simulink model "nir_d2"  (R2022a)
settings: Solver=ode15s  StartTime=0.0  StopTime=30  RelTol=1e-3
undefined symbols (not defined in the file): alpha, beta, c, dY_init, flux_init, g, Gamma, gamma_lam1, gamma_lam2, gamma_nu, gamma_Y, k, k1, k2, m, nu1, nu2, R, R_a, Y_init
settings Model: Creator=Ochir  LastModifiedBy=Ochir

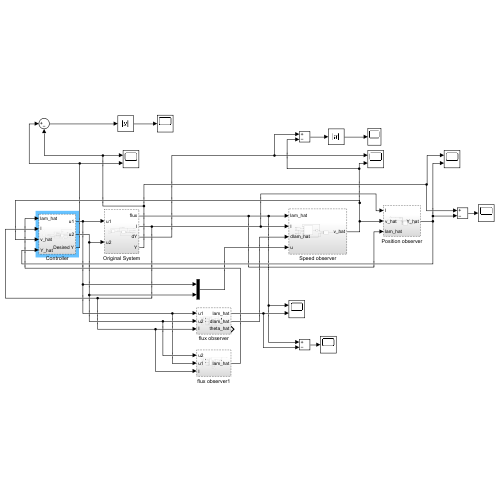
[thumbnail: Simulink's stored preview of the top-level diagram]
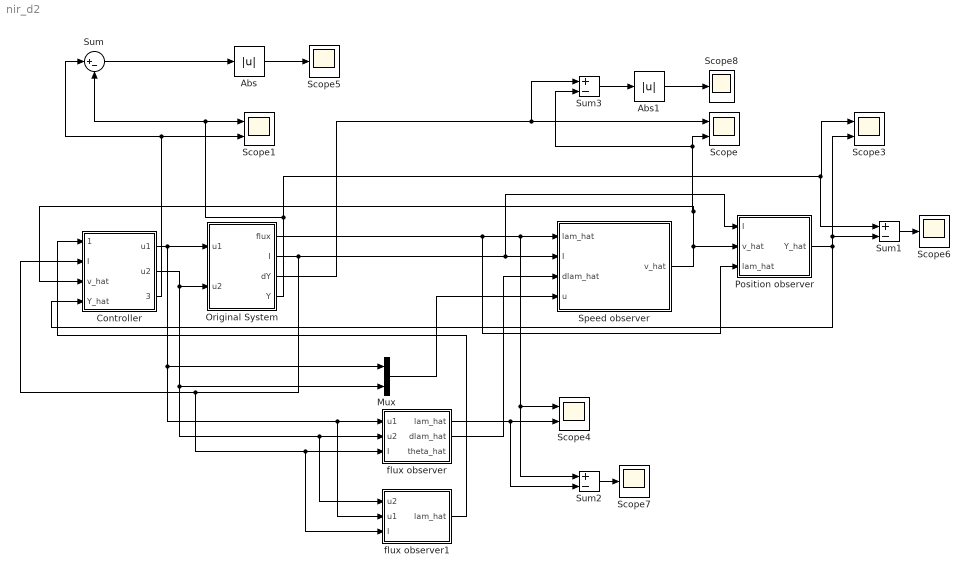
== system nir_d2 ==
  Abs : Abs  SaturateOnIntegerOverflow=off
  Abs1 : Abs  SaturateOnIntegerOverflow=off
  Controller : Subsystem  Priority=4
      settings: MinAlgLoopOccurrences=on
  Mux : Mux  Inputs=2
  Original System : Subsystem
      settings: MinAlgLoopOccurrences=on
  Position observer : Subsystem
      settings: MinAlgLoopOccurrences=on
  Scope{,1,3..4} (4 alike) : Scope  NumInputPorts=2
  Scope{5..8} (4 alike) : Scope
  Speed observer : Subsystem
      settings: MinAlgLoopOccurrences=on
  Sum : Sum  Inputs=|+-
  Sum1 : Sum  Inputs=+-
  Sum2 : Sum  Inputs=+-
  Sum3 : Sum  Inputs=+-
  flux observer : Subsystem
      settings: MinAlgLoopOccurrences=on
  flux observer1 : Subsystem
      settings: MinAlgLoopOccurrences=on
  wires:
  Controller/2(u2) -> flux observer1/1(u2), flux observer/2(u2), Mux/2, Original System/2(u2)
  Sum3/1 -> Abs1/1
  Sum2/1 -> Scope7/1
  Speed observer/1(v_hat) -> Controller/3(v_hat), Sum3/2, Scope/2, Position observer/2(v_hat)
  flux observer/2(dlam_hat) -> Speed observer/3(dlam_hat)
  flux observer/1(lam_hat) -> Sum2/2, Scope4/2
  Position observer/1(Y_hat) -> Controller/4(Y_hat), Sum1/2, Scope3/2
  Original System/2(I) -> Position observer/1(I), Speed observer/2(I), flux observer1/3(I), flux observer/3(I), Controller/2(I)
  flux observer1/1(lam_hat) -> Controller/1(lam_hat)
  Controller/1(u1) -> flux observer1/2(u1), flux observer/1(u1), Mux/1, Original System/1(u1)
  Abs/1 -> Scope5/1
  Original System/4(Y) -> Scope1/1, Sum/2, Sum1/1, Scope3/1
  Original System/1(flux) -> Position observer/3(lam_hat), Sum2/1, Scope4/1, Speed observer/1(lam_hat)
  Sum1/1 -> Scope6/1
  Controller/3(Desired Y) -> Scope1/2, Sum/1
  Sum/1 -> Abs/1
  Mux/1 -> Speed observer/4(u)
  Original System/3(dY) -> Sum3/1, Scope/1
  Abs1/1 -> Scope8/1

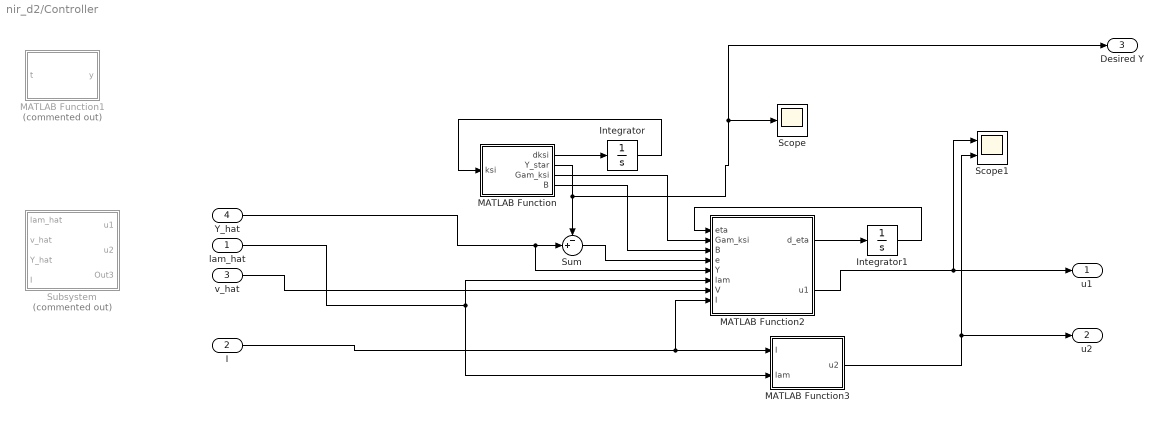
== system nir_d2/Controller ==
  lam_hat : Inport
  I : Inport  Port=2
  v_hat : Inport  Port=3
  Y_hat : Inport  Port=4
  Integrator : Integrator  InitialCondition=[0.01; -0.01]
  Integrator1 : Integrator  InitialCondition=[0.01; -0.01]
  MATLAB Function : MATLAB Function  TreatAsAtomicUnit=on
  MATLAB Function1 : MATLAB Function  Commented=on  TreatAsAtomicUnit=on
  MATLAB Function2 : MATLAB Function  TreatAsAtomicUnit=on
  MATLAB Function3 : MATLAB Function  TreatAsAtomicUnit=on
  Scope : Scope
  Scope1 : Scope  NumInputPorts=2
  Subsystem : Subsystem  Commented=on
  Sum : Sum  Inputs=-+|
  u1 : Outport
  u2 : Outport  Port=2
  Desired Y : Outport  Port=3
  wires:
  Integrator1/1 -> MATLAB Function2/1(eta)
  lam_hat/1 -> MATLAB Function3/2(lam), MATLAB Function2/6(lam)
  MATLAB Function2/1(d_eta) -> Integrator1/1
  Sum/1 -> MATLAB Function2/4(e)
  Y_hat/1 -> MATLAB Function2/5(Y), Sum/2
  Integrator/1 -> MATLAB Function/1(ksi)
  MATLAB Function/3(Gam_ksi) -> MATLAB Function2/2(Gam_ksi)
  MATLAB Function/1(dksi) -> Integrator/1
  MATLAB Function/2(Y_star) -> Sum/1, Desired Y/1, Scope/1
  MATLAB Function3/1(u2) -> u2/1, Scope1/2
  MATLAB Function2/2(u1) -> u1/1, Scope1/1
  MATLAB Function/4(B) -> MATLAB Function2/3(B)
  v_hat/1 -> MATLAB Function2/7(V)
  I/1 -> MATLAB Function2/8(I), MATLAB Function3/1(I)

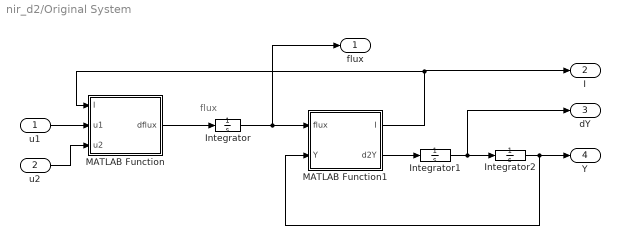
== system nir_d2/Original System ==
  note: flux
  u1 : Inport
  u2 : Inport  Port=2
  Integrator : Integrator  InitialCondition=flux_init  UpperSaturationLimit=1e12  LowerSaturationLimit=-1e12
  Integrator1 : Integrator  InitialCondition=dY_init  UpperSaturationLimit=1e12  LowerSaturationLimit=-1e12
  Integrator2 : Integrator  InitialCondition=Y_init  UpperSaturationLimit=1e12  LowerSaturationLimit=-1e12
  MATLAB Function : MATLAB Function  Priority=0
  MATLAB Function1 : MATLAB Function  Priority=0
  flux : Outport
  I : Outport  Port=2
  dY : Outport  Port=3
  Y : Outport  Port=4
  wires:
  Integrator/1 -> flux/1, MATLAB Function1/1(flux)
  u1/1 -> MATLAB Function/2(u1)
  u2/1 -> MATLAB Function/3(u2)
  MATLAB Function/1(dflux) -> Integrator/1
  MATLAB Function1/2(d2Y) -> Integrator1/1
  Integrator1/1 -> dY/1, Integrator2/1
  Integrator2/1 -> Y/1, MATLAB Function1/2(Y)
  MATLAB Function1/1(I) -> I/1, MATLAB Function/1(I)

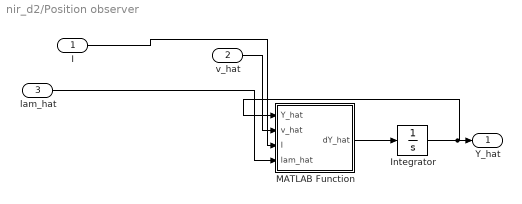
== system nir_d2/Position observer ==
  I : Inport
  v_hat : Inport  Port=2
  lam_hat : Inport  Port=3
  Integrator : Integrator  UpperSaturationLimit=1e12  LowerSaturationLimit=-1e12
  MATLAB Function : MATLAB Function
  Y_hat : Outport
  wires:
  Integrator/1 -> MATLAB Function/1(Y_hat), Y_hat/1
  lam_hat/1 -> MATLAB Function/4(lam_hat)
  I/1 -> MATLAB Function/3(I)
  v_hat/1 -> MATLAB Function/2(v_hat)
  MATLAB Function/1(dY_hat) -> Integrator/1

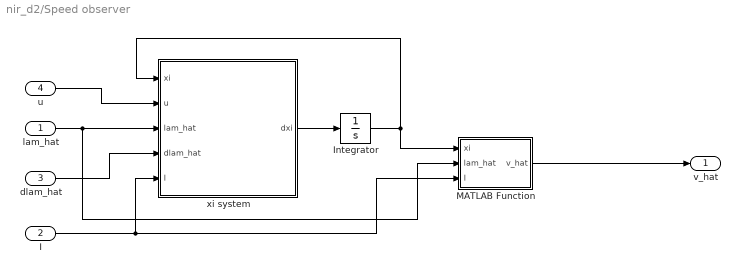
== system nir_d2/Speed observer ==
  lam_hat : Inport
  I : Inport  Port=2
  dlam_hat : Inport  Port=3
  u : Inport  Port=4
  Integrator : Integrator  UpperSaturationLimit=1e12  LowerSaturationLimit=-1e12
  MATLAB Function : MATLAB Function
  xi system : MATLAB Function
  v_hat : Outport
  wires:
  dlam_hat/1 -> xi system/4(dlam_hat)
  I/1 -> xi system/5(I), MATLAB Function/3(I)
  Integrator/1 -> xi system/1(xi), MATLAB Function/1(xi)
  xi system/1(dxi) -> Integrator/1
  MATLAB Function/1(v_hat) -> v_hat/1
  u/1 -> xi system/2(u)
  lam_hat/1 -> MATLAB Function/2(lam_hat), xi system/3(lam_hat)

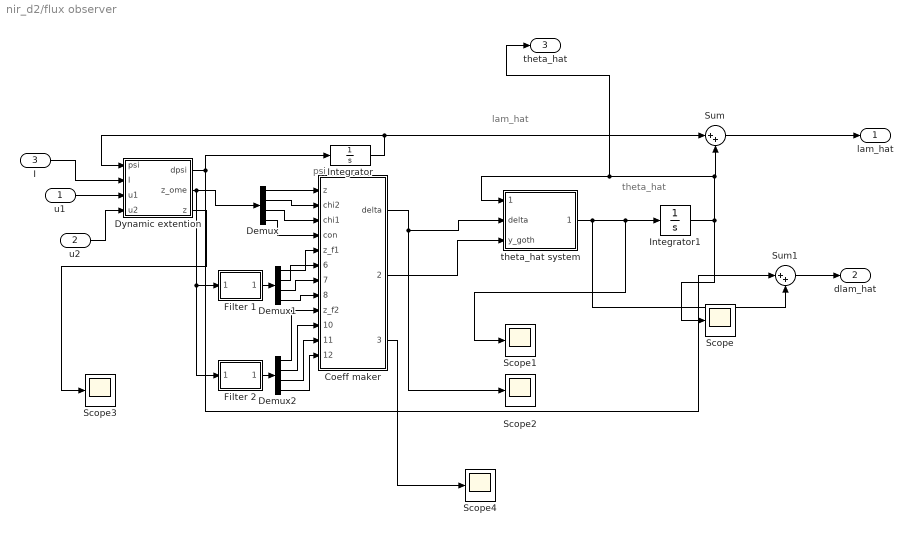
== system nir_d2/flux observer ==
  note: lam_hat
  note: theta_hat
  note: psi
  u1 : Inport
  u2 : Inport  Port=2
  I : Inport  Port=3
  Coeff maker : MATLAB Function  Priority=4
  Demux : Demux
  Demux1 : Demux
  Demux2 : Demux
  Dynamic extention : MATLAB Function  Priority=0
  Filter 1 : Subsystem  Priority=0
  Filter 2 : Subsystem  Priority=1
  Integrator : Integrator  InitialCondition=[0;0]  UpperSaturationLimit=1e12  LowerSaturationLimit=-1e12
  Integrator1 : Integrator  InitialCondition=[0;0]  UpperSaturationLimit=1e12  LowerSaturationLimit=-1e12
  Scope{,1..4} (5 alike) : Scope
  Sum : Sum  Priority=8  Inputs=|++
  Sum1 : Sum  Priority=7  Inputs=|++
  theta_hat system : MATLAB Function  Priority=5
  lam_hat : Outport
  dlam_hat : Outport  Port=2
  theta_hat : Outport  Port=3
  wires:
  u2/1 -> Dynamic extention/4(u2)
  Integrator/1 -> Dynamic extention/1(psi), Sum/1
  u1/1 -> Dynamic extention/3(u1)
  Sum/1 -> lam_hat/1
  Sum1/1 -> dlam_hat/1
  Dynamic extention/1(dpsi) -> Sum1/1, Integrator/1
  Dynamic extention/2(z_ome) -> Demux/1, Filter 2/1(z_ome), Filter 1/1(z_ome)
  I/1 -> Dynamic extention/2(I)
  theta_hat system/1(dtheta_hat) -> Sum1/2, Scope1/1, Integrator1/1
  Coeff maker/2(y_goth) -> theta_hat system/3(y_goth)
  Coeff maker/1(delta) -> Scope2/1, theta_hat system/2(delta)
  Integrator1/1 -> Scope/1, theta_hat system/1(theta_hat), theta_hat/1, Sum/2
  Demux/1 -> Coeff maker/1(z)
  Demux/2 -> Coeff maker/2(chi2)
  Demux/3 -> Coeff maker/3(chi1)
  Demux/4 -> Coeff maker/4(con)
  Filter 1/1(Output) -> Demux1/1
  Demux1/1 -> Coeff maker/5(z_f1)
  Demux1/2 -> Coeff maker/6(chi2_f1)
  Demux1/3 -> Coeff maker/7(chi1_f1)
  Demux1/4 -> Coeff maker/8(con_f1)
  Filter 2/1(Output) -> Demux2/1
  Demux2/1 -> Coeff maker/9(z_f2)
  Demux2/2 -> Coeff maker/10(chi2_f2)
  Demux2/3 -> Coeff maker/11(chi1_f2)
  Demux2/4 -> Coeff maker/12(con_f2)
  Dynamic extention/3(z) -> Scope3/1
  Coeff maker/3(rang_Omega) -> Scope4/1

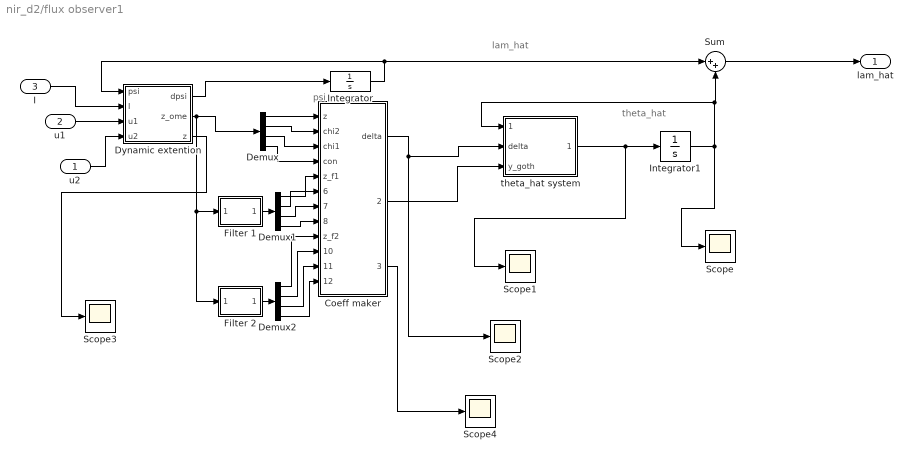
== system nir_d2/flux observer1 ==
  note: lam_hat
  note: theta_hat
  note: psi
  u2 : Inport
  u1 : Inport  Port=2
  I : Inport  Port=3
  Coeff maker : MATLAB Function  Priority=4
  Demux : Demux
  Demux1 : Demux
  Demux2 : Demux
  Dynamic extention : MATLAB Function  Priority=0
  Filter 1 : Subsystem  Priority=0
  Filter 2 : Subsystem  Priority=1
  Integrator : Integrator  InitialCondition=[0;0]  UpperSaturationLimit=1e12  LowerSaturationLimit=-1e12
  Integrator1 : Integrator  InitialCondition=[0;0]  UpperSaturationLimit=1e12  LowerSaturationLimit=-1e12
  Scope{,1..4} (5 alike) : Scope
  Sum : Sum  Priority=8  Inputs=|++
  theta_hat system : MATLAB Function  Priority=5
  lam_hat : Outport
  wires:
  u2/1 -> Dynamic extention/4(u2)
  Integrator/1 -> Dynamic extention/1(psi), Sum/1
  u1/1 -> Dynamic extention/3(u1)
  Sum/1 -> lam_hat/1
  Dynamic extention/1(dpsi) -> Integrator/1
  Dynamic extention/2(z_ome) -> Demux/1, Filter 2/1(z_ome), Filter 1/1(z_ome)
  I/1 -> Dynamic extention/2(I)
  theta_hat system/1(dtheta_hat) -> Scope1/1, Integrator1/1
  Coeff maker/2(y_goth) -> theta_hat system/3(y_goth)
  Coeff maker/1(delta) -> Scope2/1, theta_hat system/2(delta)
  Integrator1/1 -> Scope/1, theta_hat system/1(theta_hat), Sum/2
  Demux/1 -> Coeff maker/1(z)
  Demux/2 -> Coeff maker/2(chi2)
  Demux/3 -> Coeff maker/3(chi1)
  Demux/4 -> Coeff maker/4(con)
  Filter 1/1(Output) -> Demux1/1
  Demux1/1 -> Coeff maker/5(z_f1)
  Demux1/2 -> Coeff maker/6(chi2_f1)
  Demux1/3 -> Coeff maker/7(chi1_f1)
  Demux1/4 -> Coeff maker/8(con_f1)
  Filter 2/1(Output) -> Demux2/1
  Demux2/1 -> Coeff maker/9(z_f2)
  Demux2/2 -> Coeff maker/10(chi2_f2)
  Demux2/3 -> Coeff maker/11(chi1_f2)
  Demux2/4 -> Coeff maker/12(con_f2)
  Dynamic extention/3(z) -> Scope3/1
  Coeff maker/3(rang_Omega) -> Scope4/1

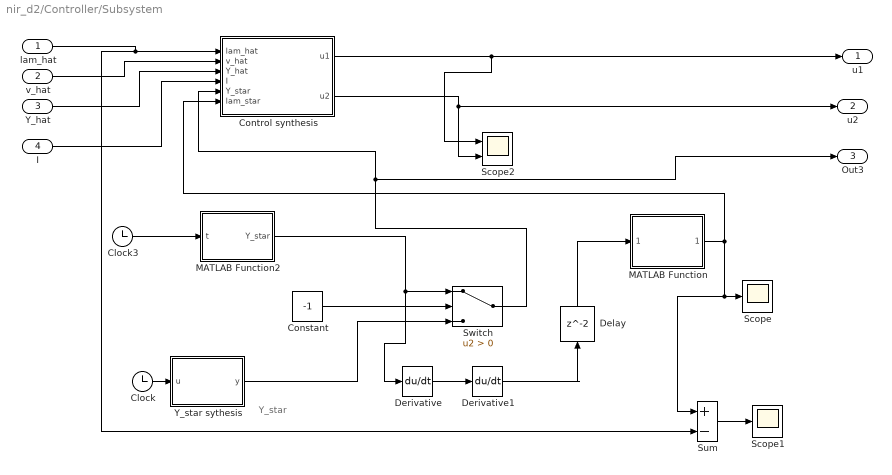
== system nir_d2/Controller/Subsystem ==
  note: Y_star
  lam_hat : Inport
  v_hat : Inport  Port=2
  Y_hat : Inport  Port=3
  I : Inport  Port=4
  Clock : Clock
  Clock3 : Clock
  Constant : Constant  Value=-1
  Control synthesis : MATLAB Function  Priority=1
  Delay : Delay
  Derivative : Derivative
  Derivative1 : Derivative
  MATLAB Function : MATLAB Function  TreatAsAtomicUnit=on
  MATLAB Function2 : MATLAB Function  TreatAsAtomicUnit=on
  Scope : Scope
  Scope1 : Scope
  Scope2 : Scope  NumInputPorts=2
  Sum : Sum  Inputs=+-
  Switch : Switch  Criteria=u2 > Threshold  SaturateOnIntegerOverflow=off  InputSameDT=off
  Y_star sythesis : MATLAB Function  Priority=0
  u1 : Outport
  u2 : Outport  Port=2
  Out3 : Outport  Port=3
  wires:
  MATLAB Function2/1(Y_star) -> Derivative/1, Switch/1
  MATLAB Function/1(lambda_star) -> Scope/1, Sum/1, Control synthesis/6(lam_star)
  lam_hat/1 -> Control synthesis/1(lam_hat), Sum/2
  Clock/1 -> Y_star sythesis/1(u)
  Y_star sythesis/1(y) -> Switch/3
  Switch/1 -> Out3/1, Control synthesis/5(Y_star)
  Constant/1 -> Switch/2
  Derivative/1 -> Derivative1/1
  Clock3/1 -> MATLAB Function2/1(t)
  Control synthesis/2(u2) -> u2/1, Scope2/2
  Control synthesis/1(u1) -> u1/1, Scope2/1
  Derivative1/1 -> Delay/1
  Sum/1 -> Scope1/1
  Delay/1 -> MATLAB Function/1(d2Y_star)
  v_hat/1 -> Control synthesis/2(v_hat)
  Y_hat/1 -> Control synthesis/3(Y_hat)
  I/1 -> Control synthesis/4(I)

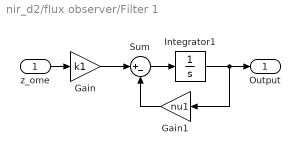
== system nir_d2/flux observer/Filter 1 ==
  z_ome : Inport
  Gain : Gain  Gain=k1
  Gain1 : Gain  Gain=nu1
  Integrator1 : Integrator  InitialCondition=[0; 0; 0; 0]  UpperSaturationLimit=1e12  LowerSaturationLimit=-1e12
  Sum : Sum  Inputs=|+-
  Output : Outport
  wires:
  Sum/1 -> Integrator1/1
  Gain/1 -> Sum/1
  Integrator1/1 -> Output/1, Gain1/1
  Gain1/1 -> Sum/2
  z_ome/1 -> Gain/1

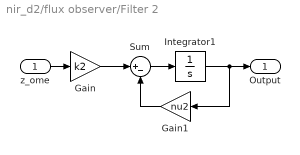
== system nir_d2/flux observer/Filter 2 ==
  z_ome : Inport
  Gain : Gain  Gain=k2
  Gain1 : Gain  Gain=nu2
  Integrator1 : Integrator  InitialCondition=[0; 0; 0; 0]  UpperSaturationLimit=1e12  LowerSaturationLimit=-1e12
  Sum : Sum  Inputs=|+-
  Output : Outport
  wires:
  Sum/1 -> Integrator1/1
  Gain/1 -> Sum/1
  Integrator1/1 -> Output/1, Gain1/1
  Gain1/1 -> Sum/2
  z_ome/1 -> Gain/1

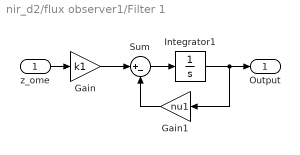
== system nir_d2/flux observer1/Filter 1 ==
  z_ome : Inport
  Gain : Gain  Gain=k1
  Gain1 : Gain  Gain=nu1
  Integrator1 : Integrator  InitialCondition=[0; 0; 0; 0]  UpperSaturationLimit=1e12  LowerSaturationLimit=-1e12
  Sum : Sum  Inputs=|+-
  Output : Outport
  wires:
  Sum/1 -> Integrator1/1
  Gain/1 -> Sum/1
  Integrator1/1 -> Output/1, Gain1/1
  Gain1/1 -> Sum/2
  z_ome/1 -> Gain/1

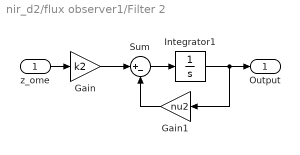
== system nir_d2/flux observer1/Filter 2 ==
  z_ome : Inport
  Gain : Gain  Gain=k2
  Gain1 : Gain  Gain=nu2
  Integrator1 : Integrator  InitialCondition=[0; 0; 0; 0]  UpperSaturationLimit=1e12  LowerSaturationLimit=-1e12
  Sum : Sum  Inputs=|+-
  Output : Outport
  wires:
  Sum/1 -> Integrator1/1
  Gain/1 -> Sum/1
  Integrator1/1 -> Output/1, Gain1/1
  Gain1/1 -> Sum/2
  z_ome/1 -> Gain/1

== matlab function nir_d2/Controller/Subsystem/Control synthesis ==
  data: lam_hat input size=[2,1]; u1 output size=1; v_hat input size=1; Y_hat input size=1; I input size=[2,1]; Y_star input size=1; u2 output size=1; R parameter; k parameter; alpha parameter; beta parameter; Gamma parameter; m parameter; R_a parameter; lam_star input
function [u1, u2] = fcn(lam_hat, v_hat, Y_hat, I, Y_star, R, k, alpha, beta, Gamma, m, R_a, lam_star)
    lam_wave = [0;0];
    lam_wave(1) = (lam_hat(1) - lam_star(1));
    lam_wave(2) = lam_hat(2) - lam_star(2);
    Y_wave = (Y_hat - Y_star);
    u1 = R*I(1) - R/2/k/alpha*(lam_hat(1)^2 - lam_star(1)^2) - (R/alpha+alpha*R_a)*...
          Gamma*(1/alpha*lam_wave(1) + Y_wave + R_a*m*v_hat) - alpha*v_hat;
    
    u2 = R*I(2) - R/2/k/beta*(lam_hat(2)^2 - lam_star(2)^2) + beta*R_a*...
          Gamma*(1/alpha*lam_wave(1) + Y_wave + R_a*m*v_hat) + beta*v_hat;

== matlab function nir_d2/flux observer1/Dynamic extention ==
  data: psi input size=[2,1]; I input size=[2,1]; dpsi output size=[2, 1]; u1 input; u2 input; g parameter; c parameter; m parameter; k parameter; R parameter; z_ome output; z output size=1
function [dpsi, z_ome, z]  = fcn(psi, I, u1, u2, g, c, m, k, R)
    u = [u1; u2];
    dpsi = -R*I + u;
    z = -I(1)*psi(2)-I(2)*psi(1) + 2*c/k*psi(1)*psi(2);
    chi = I - 2*c/k*psi;
    
    z_ome = [z; chi(2); chi(1); -(2*c/k)];

== matlab function nir_d2/flux observer1/theta_hat system ==
  data: theta_hat input; delta input; y_goth input; dtheta_hat output size=[2, 1]; gamma_lam1 parameter; gamma_lam2 parameter
function dtheta_hat = fcn(theta_hat, delta, y_goth, gamma_lam1, gamma_lam2)
 
    dtheta_hat = [gamma_lam1*delta*(y_goth(1) - delta*theta_hat(1)); ...
                gamma_lam2*delta*(y_goth(2) - delta*theta_hat(2))];

== matlab function nir_d2/Controller/Subsystem/MATLAB Function ==
  data: d2Y_star input; lambda_star output; k parameter; m parameter; g parameter
function lambda_star = fcn(d2Y_star, k, m, g)

    lambda_star = [0; 0];
    lambda_star(2) = 1;
    lambda_star(1) = sqrt(2*k*m*(g+0) + 1^2);
    %lambda_star(1) = sqrt(2*k*m*g + 1);

== matlab function nir_d2/Original System/MATLAB Function ==
  data: I input; dflux output size=[2 1]; u1 input; u2 input; R parameter
function dflux  = fcn(I, u1, u2, R)
    dflux = [-R*I(1) + u1; -R*I(2) + u2];

== matlab function nir_d2/Speed observer/xi system ==
  data: xi input; dxi output size=1; u input; lam_hat input; dlam_hat input; I input; g parameter; k parameter; m parameter; gamma_nu parameter; R parameter
function dxi = fcn(xi, u, lam_hat, dlam_hat, I, g, k, m, gamma_nu, R)
    dlam = -R*I + u;
    dxi = -gamma_nu*(norm(lam_hat)^2)*(xi - gamma_nu*k*( I(1)*lam_hat(1) -I(2)*lam_hat(2)))...
         + gamma_nu*k*I(1)*(dlam(1) + dlam_hat(1)) - gamma_nu*k*I(2)*(dlam(2) + dlam_hat(2))...
          + 1/2/k/m*((lam_hat(1))^2 - (lam_hat(2))^2) - g;

    

    %dxi = -gamma_nu*(norm(lam)^2*v_hat - 2*k*(I(1)*dlam(1) - I(2)*dlam(2))) + 1/2/k/m*(lam(1)^2-lam(2)^2-2*k*m*g);

== matlab function nir_d2/Position observer/MATLAB Function ==
  data: Y_hat input; dY_hat output size=1; v_hat input; I input; lam_hat input; gamma_Y parameter; k parameter; c parameter
function dY_hat = fcn(Y_hat, v_hat, I, lam_hat, gamma_Y, k, c)

    dY_hat = v_hat - gamma_Y*(norm(lam_hat)^2*Y_hat + (k*I(1) - c*lam_hat(1))*lam_hat(1) ...
              - (k*I(2) - c*lam_hat(2))*lam_hat(2));

== matlab function nir_d2/Controller/Subsystem/Y_star sythesis ==
  data: u input; y output
function y = fcn(u)
    f = 0;
    if (u>=0) && (u<1)
        f = 0.001;
    end
    if (u>=1) && (u<2)
        f = 0.002;
    end
    if (u>=2) && (u<3)
        f = -0.001;
    end
    if (u>=3) && (u<4)
        f = 0.001;
    end
    if (u>=4) && (u<5)
        f = 0.003;
    end
    if (u>=5)
        f = 0.001;
    end
    y = f;

== matlab function nir_d2/Speed observer/MATLAB Function ==
  data: xi input; v_hat output; lam_hat input; I input; gamma_nu parameter; k parameter
function v_hat = fcn(xi, lam_hat, I, gamma_nu, k)

    v_hat = xi - gamma_nu*k*(I(1)*lam_hat(1) - I(2)*lam_hat(2));

== matlab function nir_d2/Controller/MATLAB Function1 ==
  data: t input; y output
function y = fcn(t)

y = -0.005*sin(0.5*t) - 0.05*sin(t) + 0.1575*sin(1.5*t);

== matlab function nir_d2/Original System/MATLAB Function1 ==
  data: I output; flux input; g parameter; m parameter; k parameter; d2Y output; Y input; c parameter
function [I, d2Y]  = fcn(flux, g, m, k, Y, c)
    lam1 = flux(1);
    lam2 = flux(2);
    d2Y = 1/2/k/m*(lam1.^2-lam2.^2) - g;
    I = [1/k*(c - Y)*lam1; 1/k*(c + Y)*lam2];

== matlab function nir_d2/Controller/Subsystem/MATLAB Function2 ==
  data: t input; Y_star output
function Y_star = fcn(t)

Y_star = 0.02*sin(0.5*t) + 0.05*sin(t) - 0.07*sin(1.5*t);

== matlab function nir_d2/Controller/MATLAB Function ==
  data: ksi input; dksi output; Y_star output; Gam_ksi output; B output
function [dksi, Y_star, Gam_ksi, B] = fcn(ksi)

Gam_ksi = [0 2; -2 0];
%Gam_ksi = -eye(2);
B = [1; 1];
H_ksi = [1 1];
dksi = Gam_ksi*ksi;
Y_star = H_ksi*ksi;

== matlab function nir_d2/Controller/MATLAB Function2 ==
  data: eta input; Gam_ksi input; B input; e input; d_eta output; Y input; lam input size=[2, 1]; V input; R parameter; I input; u1 output; k parameter; c parameter
function [d_eta, u1] = fcn(eta, Gam_ksi, B, e, Y, lam, V, R, I, k, c)
%B = [1; 1];
d_eta = Gam_ksi*eta + B*e;

k1 = 500; % 3000 %
k_eta = 300*[1 1]; % 0.01*[1 -1]
k2 = -300; % -10 or -20
k3 = R/k*(c-Y);
u1 = k1*e + k_eta*eta - k2*V - k3*lam(2);
%k1_2 = 10;
%k_eta_2 = 0.001*[1 -1];
%k2_2 = 100;
%k3_2 = R/k*(c+Y);
%u2 = k1_2*e + k_eta_2*eta - k2_2*V - k3_2*lam(1);

== matlab function nir_d2/Controller/MATLAB Function3 ==
  data: I input size=[2, 1]; u2 output; R parameter; lam input
function u2 = fcn(I, R, lam)

u2 = I(2)*R + (2 - lam(2));

== matlab function nir_d2/flux observer1/Coeff maker ==
  data: z input; chi2 input; chi1 input; con input; delta output size=1; z_f1 input; chi2_f1 input; chi1_f1 input; con_f1 input; z_f2 input; chi2_f2 input; y_goth output size=[3, 1]; chi1_f2 input; con_f2 input; rang_Omega output
function [delta, y_goth, rang_Omega] = fcn(z, chi2, chi1, con, z_f1, chi2_f1, chi1_f1, con_f1, z_f2, chi2_f2, chi1_f2, con_f2)
    
    Z = [z; z_f1; z_f2];
    Omega = [chi2, chi1, con; chi2_f1, chi1_f1, con_f1; chi2_f2, chi1_f2, con_f2];
    delta = det(Omega);
    adj = eye(3, 3);

    adj(1, 1) = det([Omega(2, 2) Omega(2, 3); Omega(3, 2) Omega(3, 3)]);
    adj(1, 2) = -det([Omega(2, 1) Omega(2, 3); Omega(3, 1) Omega(3, 3)]);
    adj(1, 3) = det([Omega(2, 1) Omega(2, 2); Omega(3, 1) Omega(3, 2)]);

    adj(2, 1) = -det([Omega(1, 2) Omega(1, 3); Omega(3, 2) Omega(3, 3)]);
    adj(2, 2) = det([Omega(1, 1) Omega(1, 3); Omega(3, 1) Omega(3, 3)]);
    adj(2, 3) = -det([Omega(1, 1) Omega(1, 2); Omega(3, 1) Omega(3, 2)]);

    adj(3, 1) = det([Omega(1, 2) Omega(1, 3); Omega(2, 2) Omega(2, 3)]);
    adj(3, 2) = -det([Omega(1, 1) Omega(1, 3); Omega(2, 1) Omega(2, 3)]);
    adj(3, 3) = det([Omega(1, 1) Omega(1, 2); Omega(2, 1) Omega(2, 2)]);

    adj = adj';

    y_goth = adj*Z;

    %if norm(delta) < 1e-12
    %    delta = 0;
    %end
    rang_Omega = rank(Omega); 
    %should_be_diag = Omega*adj
    %delta

== matlab function nir_d2/flux observer/Coeff maker ==
  data: z input; chi2 input; chi1 input; con input; delta output size=1; z_f1 input; chi2_f1 input; chi1_f1 input; con_f1 input; z_f2 input; chi2_f2 input; y_goth output size=[3, 1]; chi1_f2 input; con_f2 input; rang_Omega output
function [delta, y_goth, rang_Omega] = fcn(z, chi2, chi1, con, z_f1, chi2_f1, chi1_f1, con_f1, z_f2, chi2_f2, chi1_f2, con_f2)
    
    Z = [z; z_f1; z_f2];
    Omega = [chi2, chi1, con; chi2_f1, chi1_f1, con_f1; chi2_f2, chi1_f2, con_f2];
    delta = det(Omega);
    adj = eye(3, 3);

    adj(1, 1) = det([Omega(2, 2) Omega(2, 3); Omega(3, 2) Omega(3, 3)]);
    adj(1, 2) = -det([Omega(2, 1) Omega(2, 3); Omega(3, 1) Omega(3, 3)]);
    adj(1, 3) = det([Omega(2, 1) Omega(2, 2); Omega(3, 1) Omega(3, 2)]);

    adj(2, 1) = -det([Omega(1, 2) Omega(1, 3); Omega(3, 2) Omega(3, 3)]);
    adj(2, 2) = det([Omega(1, 1) Omega(1, 3); Omega(3, 1) Omega(3, 3)]);
    adj(2, 3) = -det([Omega(1, 1) Omega(1, 2); Omega(3, 1) Omega(3, 2)]);

    adj(3, 1) = det([Omega(1, 2) Omega(1, 3); Omega(2, 2) Omega(2, 3)]);
    adj(3, 2) = -det([Omega(1, 1) Omega(1, 3); Omega(2, 1) Omega(2, 3)]);
    adj(3, 3) = det([Omega(1, 1) Omega(1, 2); Omega(2, 1) Omega(2, 2)]);

    adj = adj';

    y_goth = adj*Z;

    %if norm(delta) < 1e-12
    %    delta = 0;
    %end
    rang_Omega = rank(Omega); 
    %should_be_diag = Omega*adj
    %delta

== matlab function nir_d2/flux observer/Dynamic extention ==
  data: psi input size=[2,1]; I input size=[2,1]; dpsi output size=[2, 1]; u1 input; u2 input; g parameter; c parameter; m parameter; k parameter; R parameter; z_ome output; z output size=1
function [dpsi, z_ome, z]  = fcn(psi, I, u1, u2, g, c, m, k, R)
    u = [u1; u2];
    dpsi = -R*I + u;
    z = -I(1)*psi(2)-I(2)*psi(1) + 2*c/k*psi(1)*psi(2);
    chi = I - 2*c/k*psi;
    
    z_ome = [z; chi(2); chi(1); -(2*c/k)];

== matlab function nir_d2/flux observer/theta_hat system ==
  data: theta_hat input; delta input; y_goth input; dtheta_hat output size=[2, 1]; gamma_lam1 parameter; gamma_lam2 parameter
function dtheta_hat = fcn(theta_hat, delta, y_goth, gamma_lam1, gamma_lam2)
 
    dtheta_hat = [gamma_lam1*delta*(y_goth(1) - delta*theta_hat(1)); ...
                gamma_lam2*delta*(y_goth(2) - delta*theta_hat(2))];
